simulink model "multi_rotor_sim"  (R2023b)
settings: Solver=ode4  StartTime=0.0  StopTime=inf  FixedStep=ST  RelTol=1e-3
values from neighbouring files (symbols this model uses):
  a0 = 0    [parameters.m]
  ASLOPE = 5.9    [parameters.m]
  Ax = 0.023    [parameters.m]
  Ay = 0.023    [parameters.m]
  Az = 0.106    [parameters.m]
  BLADES = 2    [parameters.m]
  BLCG = 0    [parameters.m]
  BLCP = 0    [parameters.m]
  BLH1 = b*sind(30)    [parameters.m]
  BLH2 = b    (= 0.275)    [parameters.m]
  BLH3 = b*sind(30)    [parameters.m]
  BLH4 = -b*sind(30)    [parameters.m]
  BLH5 = -b    (= -0.275)    [parameters.m]
  BLH6 = -b*sind(30)    [parameters.m]
  chi1 = 1    [parameters.m]
  chi2 = -1    [parameters.m]
  chi3 = 1    [parameters.m]
  chi4 = -1    [parameters.m]
  chi5 = 1    [parameters.m]
  chi6 = -1    [parameters.m]
  CHORD = 17.55e-3    (= 0.01755)    [parameters.m]
  CHORD75 = 21e-3    (= 0.021)    [parameters.m]
  dyn_viscosity = 17.89e-6    (= 1.789e-05)    [parameters.m]
  g0 = 9.80665    [parameters.m]
  href = 0    [parameters.m]
  k_ind = 1.35    [parameters.m]
  k_Omega = 14.92    [parameters.m]
  latref = 44.200626    [parameters.m]
  lonref = 12.063822    [parameters.m]
  m = 2.15    [parameters.m]
  MC_ATT_PITCH = 45*pi/180    (= 0.785398163397)    [parameters.m]
  MC_ATT_ROLL = 45*pi/180    (= 0.785398163397)    [parameters.m]
  MC_PITCH_P = 2    [parameters.m]
  MC_PITCHRATE_D = 0    [parameters.m]
  MC_PITCHRATE_I = 0.05    [parameters.m]
  MC_PITCHRATE_P = 0.09*3    (= 0.27)    [parameters.m]
  MC_RATE_PITCH = 500*pi/180    (= 8.72664625997)    [parameters.m]
  MC_RATE_ROLL = 500*pi/180    (= 8.72664625997)    [parameters.m]
  MC_RATE_YAW = 300*pi/180    (= 5.23598775598)    [parameters.m]
  MC_ROLL_P = 2    [parameters.m]
  MC_ROLLRATE_D = 0    [parameters.m]
  MC_ROLLRATE_I = 0.05    [parameters.m]
  MC_ROLLRATE_P = 0.09*3    (= 0.27)    [parameters.m]
  MC_VEL_FWD = 15    [parameters.m]
  MC_VEL_FWD_OPT = 0.5    [parameters.m]
  MC_VEL_LAT = 15    [parameters.m]
  MC_VEL_LAT_OPT = 0.5    [parameters.m]
  MC_VEL_VERT = 15    [parameters.m]
  MC_YAW_P = 0.55    [parameters.m]
  MC_YAWRATE_D = 0.05    [parameters.m]
  MC_YAWRATE_I = 0.02    [parameters.m]
  MC_YAWRATE_P = 0.15*3    (= 0.45)    [parameters.m]
  MPC_XY_VEL_D_ACC = 0.6    [parameters.m]
  MPC_XY_VEL_I_ACC = 0.8    [parameters.m]
  MPC_XY_VEL_P_ACC = 1.7    [parameters.m]
  MPC_Z_VEL_D_ACC = 0    [parameters.m]
  MPC_Z_VEL_I_ACC = 2    [parameters.m]
  MPC_Z_VEL_P_ACC = 4    [parameters.m]
  n = 0.6359    [parameters.m]
  p00 = 7.145e-2    (= 0.07145)    [parameters.m]
  p01 = 0.4377    [parameters.m]
  p02 = -10.13    [parameters.m]
  p10 = 1.259e-3    (= 0.001259)    [parameters.m]
  p11 = 1.284e-3    (= 0.001284)    [parameters.m]
  p20 = -7.513e-7    (= -7.513e-07)    [parameters.m]
  PWM_hover = (PWM_idle+PWM_max)/2    (= 1550)    [parameters.m]
  PWM_idle = 1100    [parameters.m]
  PWM_max = 2000    [parameters.m]
  ROTOR = 4*0.0254    (= 0.1016)    [parameters.m]
  ST = 0.01    [parameters.m]
  STACG = 0    [parameters.m]
  STACP = 0    [parameters.m]
  STAH1 = -b*cosd(30)    [parameters.m]
  STAH2 = 0    [parameters.m]
  STAH3 = b*cosd(30)    [parameters.m]
  STAH4 = b*cosd(30)    [parameters.m]
  STAH5 = 0    [parameters.m]
  STAH6 = -b*cosd(30)    [parameters.m]
  TERMINAL_SPEED = 0.5    [parameters.m]
  Theta0 = 45*pi/180    (= 0.785398163397)    [parameters.m]
  THETT = -38.0973*pi/180    (= -0.66492332112)    [parameters.m]
  wind_rate = [ 0 0 0 ]'    [parameters.m]
  wind_velocity_e = [ 0 0 0 ]'    [parameters.m]
  WLCG = -0.02    [parameters.m]
  WLCP = -0.08    [parameters.m]
  WLH1 = 32e-3    (= 0.032)    [parameters.m]
  WLH2 = 32e-3    (= 0.032)    [parameters.m]
  WLH3 = 32e-3    (= 0.032)    [parameters.m]
  WLH4 = 32e-3    (= 0.032)    [parameters.m]
  WLH5 = 32e-3    (= 0.032)    [parameters.m]
  WLH6 = 32e-3    (= 0.032)    [parameters.m]
undefined symbols (not defined in the file or in its folder): Earth, WGS84, X, Y, Z
libraries: sm_lib x258, slpidlib x36, nesl_utility x15, sharedtransform x13, aerolibutil x4, aerolibanimutils x3, sharedutil x2, sim3dlib x1, uavsim3dlib x1, shared6dof x1, aerolibtransform2 x1, aerolibatmos2 x1
(part 11 of 11)

== matlab function multi_rotor_sim/MULTIROTOR MODEL/ROTORS FORCE AND MOMENT/ROTOR5/MATLAB Function ==
  data: BLADES input; Mrotor output; ASLOPE input; CHORD input; CHORD75 input; ROTOR input; a0 input; Theta0 input; THETT input; dyn_viscosity input; k_ind input; STACG input; BLCG input; WLCG input; STAH input; BLH input; WLH input; chi input; rho input; TAS input; omega_TAS input; Frotor output; Q output; omega input; Omega input
function [Mrotor,Frotor,Q] = fcn(BLADES,ASLOPE,CHORD,CHORD75,ROTOR,a0,Theta0,THETT,dyn_viscosity,k_ind,STACG,BLCG,WLCG,STAH,BLH,WLH,chi,rho,TAS,omega_TAS,omega,Omega)

%% preliminary calculations
A = pi*ROTOR^2; % area of rotor disc 
sigma = BLADES*CHORD/(pi*ROTOR); % solidity of rotor 
lever_arm_H = [STACG-STAH BLH-BLCG WLCG-WLH]'; % vector from cg to rotor hub
TAS_H = [1 chi 1]'.*(TAS + cross(omega_TAS,lever_arm_H)); % wind speed at rotor
uH = TAS_H(1);
vH = TAS_H(2);
wH = TAS_H(3);
beta_w = atan2(vH,uH); % sideslip angle 
Mu = sqrt(uH^2+vH^2)/(Omega*ROTOR); % advance ratio
p = omega(1); % roll rate
q = omega(2); % pitch rate
pH = chi*p;
qH = q;

%% thrust calculation

lambda = fzero(@(x) x-wH/(Omega*ROTOR)+0.5*((0.5*BLADES*rho*ASLOPE*CHORD*ROTOR*(Omega*ROTOR)^2*(x/2+ ...
         +Theta0*(1/3+Mu^2/2)+THETT*(1/4+Mu^2/4)+Mu/4*(pH/Omega*cos(beta_w)+ ...
         +qH/Omega*sin(beta_w))))/(rho*A*(Omega*ROTOR)^2))/sqrt(Mu^2+x^2), -0.1);
vi = wH-lambda*Omega*ROTOR;
T = (0.5*BLADES*rho*ASLOPE*CHORD*ROTOR*(Omega*ROTOR)^2*(lambda/2+Theta0*(1/3+Mu^2/2)+ ...
    +THETT*(1/4+Mu^2/4)+Mu/4*(pH/Omega*cos(beta_w)+qH/Omega*sin(beta_w))));
CT = T/(rho*A*(Omega*ROTOR)^2);
V75 = sqrt(vi^2+(0.75*(Omega*ROTOR))^2);
Re = rho*CHORD75*V75/dyn_viscosity;
delta = 0.1166*Re^(-0.2)+0.3/ASLOPE^2*(6*CT/sigma/(1+3/2*Mu^2))^2;

%% forces and moments in the hub-wind frame

H_w = BLADES/2*rho*ASLOPE*CHORD*ROTOR*(Omega*ROTOR)^2*(delta*Mu/(2*ASLOPE)-1/4*Theta0*(2*lambda*Mu+ ...
      +2/3*(pH/Omega*cos(beta_w)+qH/Omega*sin(beta_w)))-THETT/4*(Mu*lambda+1/2*(pH/Omega*cos(beta_w)+ ...
      +qH/Omega*sin(beta_w)))+1/4*(-2*a0/3*(-pH/Omega*sin(beta_w)+qH/Omega*cos(beta_w))+ ...
      -2*lambda*(pH/Omega*cos(beta_w)+qH/Omega*sin(beta_w)))+Mu/4*a0^2);
Y_w = BLADES/2*rho*ASLOPE*CHORD*ROTOR*(Omega*ROTOR)^2*(-1/4*Theta0*(3*a0*Mu+ ...
      -2/3*(-pH/Omega*sin(beta_w)+qH/Omega*cos(beta_w)))-THETT/4*(2*a0*Mu+ ...
      -1/2*(-pH/Omega*sin(beta_w)+qH/Omega*cos(beta_w)))-1/4*(2*a0/3*(pH/Omega*cos(beta_w)+ ...
      +qH/Omega*sin(beta_w))-2*lambda*(-pH/Omega*sin(beta_w)+qH/Omega*cos(beta_w)))-Mu/4*6*a0*lambda);
L_w = 0;
M_w = 0;
Q = k_ind*BLADES/2*rho*ASLOPE*CHORD*ROTOR^2*(Omega*ROTOR)^2*(delta/k_ind/(4*ASLOPE)*(1+Mu^2)-Theta0*(lambda/3+ ...
    +Mu/6*(pH/Omega*cos(beta_w)+qH/Omega*sin(beta_w)))-THETT*lambda/4-1/2*lambda^2+ ...
    +Mu/3*a0*(-pH/Omega*sin(beta_w)+qH/Omega*cos(beta_w))-1/8*(-pH/Omega*sin(beta_w)+ ...
    +qH/Omega*cos(beta_w))^2-1/8*(pH/Omega*cos(beta_w)+qH/Omega*sin(beta_w))^2);


%% back rotation from hub_wind frame to hub-frame

H_H = H_w*cos(beta_w)+Y_w*sin(beta_w);
Y_H = -H_w*sin(beta_w)+Y_w*cos(beta_w);
L_H = L_w*cos(beta_w)-M_w*sin(beta_w);
M_H = L_w*sin(beta_w)+M_w*cos(beta_w);

%% back rotation from hub-frame to body-frame

X = -H_H;
Y = chi*Y_H;
Z = -T;
Frotor = [X Y Z]';
Mrotor = [chi*L_H M_H chi*Q]'+cross(lever_arm_H,Frotor);

== matlab function multi_rotor_sim/MULTIROTOR MODEL/ROTORS FORCE AND MOMENT/ROTOR6/ELECTRICAL EFFICIENCY MODEL ==
  data: Q input; Pe output; Omega input; p00 input; p10 input; p01 input; p20 input; p11 input; p02 input
function Pe = fcn(Q,Omega,p00,p10,p01,p20,p11,p02)
eta_e = p00 + p10*Omega + p01*Q + p20*Omega^2 + p02*Q^2 + p11*Omega*Q;
Psh = Omega*Q;
Pe = Psh/eta_e;

== matlab function multi_rotor_sim/MULTIROTOR MODEL/ROTORS FORCE AND MOMENT/ROTOR6/MATLAB Function ==
  data: BLADES input; Mrotor output; ASLOPE input; CHORD input; CHORD75 input; ROTOR input; a0 input; Theta0 input; THETT input; dyn_viscosity input; k_ind input; STACG input; BLCG input; WLCG input; STAH input; BLH input; WLH input; chi input; rho input; TAS input; omega_TAS input; Frotor output; Q output; omega input; Omega input
function [Mrotor,Frotor,Q] = fcn(BLADES,ASLOPE,CHORD,CHORD75,ROTOR,a0,Theta0,THETT,dyn_viscosity,k_ind,STACG,BLCG,WLCG,STAH,BLH,WLH,chi,rho,TAS,omega_TAS,omega,Omega)

%% preliminary calculations
A = pi*ROTOR^2; % area of rotor disc 
sigma = BLADES*CHORD/(pi*ROTOR); % solidity of rotor 
lever_arm_H = [STACG-STAH BLH-BLCG WLCG-WLH]'; % vector from cg to rotor hub
TAS_H = [1 chi 1]'.*(TAS + cross(omega_TAS,lever_arm_H)); % wind speed at rotor
uH = TAS_H(1);
vH = TAS_H(2);
wH = TAS_H(3);
beta_w = atan2(vH,uH); % sideslip angle 
Mu = sqrt(uH^2+vH^2)/(Omega*ROTOR); % advance ratio
p = omega(1); % roll rate
q = omega(2); % pitch rate
pH = chi*p;
qH = q;

%% thrust calculation

lambda = fzero(@(x) x-wH/(Omega*ROTOR)+0.5*((0.5*BLADES*rho*ASLOPE*CHORD*ROTOR*(Omega*ROTOR)^2*(x/2+ ...
         +Theta0*(1/3+Mu^2/2)+THETT*(1/4+Mu^2/4)+Mu/4*(pH/Omega*cos(beta_w)+ ...
         +qH/Omega*sin(beta_w))))/(rho*A*(Omega*ROTOR)^2))/sqrt(Mu^2+x^2), -0.1);
vi = wH-lambda*Omega*ROTOR;
T = (0.5*BLADES*rho*ASLOPE*CHORD*ROTOR*(Omega*ROTOR)^2*(lambda/2+Theta0*(1/3+Mu^2/2)+ ...
    +THETT*(1/4+Mu^2/4)+Mu/4*(pH/Omega*cos(beta_w)+qH/Omega*sin(beta_w))));
CT = T/(rho*A*(Omega*ROTOR)^2);
V75 = sqrt(vi^2+(0.75*(Omega*ROTOR))^2);
Re = rho*CHORD75*V75/dyn_viscosity;
delta = 0.1166*Re^(-0.2)+0.3/ASLOPE^2*(6*CT/sigma/(1+3/2*Mu^2))^2;

%% forces and moments in the hub-wind frame

H_w = BLADES/2*rho*ASLOPE*CHORD*ROTOR*(Omega*ROTOR)^2*(delta*Mu/(2*ASLOPE)-1/4*Theta0*(2*lambda*Mu+ ...
      +2/3*(pH/Omega*cos(beta_w)+qH/Omega*sin(beta_w)))-THETT/4*(Mu*lambda+1/2*(pH/Omega*cos(beta_w)+ ...
      +qH/Omega*sin(beta_w)))+1/4*(-2*a0/3*(-pH/Omega*sin(beta_w)+qH/Omega*cos(beta_w))+ ...
      -2*lambda*(pH/Omega*cos(beta_w)+qH/Omega*sin(beta_w)))+Mu/4*a0^2);
Y_w = BLADES/2*rho*ASLOPE*CHORD*ROTOR*(Omega*ROTOR)^2*(-1/4*Theta0*(3*a0*Mu+ ...
      -2/3*(-pH/Omega*sin(beta_w)+qH/Omega*cos(beta_w)))-THETT/4*(2*a0*Mu+ ...
      -1/2*(-pH/Omega*sin(beta_w)+qH/Omega*cos(beta_w)))-1/4*(2*a0/3*(pH/Omega*cos(beta_w)+ ...
      +qH/Omega*sin(beta_w))-2*lambda*(-pH/Omega*sin(beta_w)+qH/Omega*cos(beta_w)))-Mu/4*6*a0*lambda);
L_w = 0;
M_w = 0;
Q = k_ind*BLADES/2*rho*ASLOPE*CHORD*ROTOR^2*(Omega*ROTOR)^2*(delta/k_ind/(4*ASLOPE)*(1+Mu^2)-Theta0*(lambda/3+ ...
    +Mu/6*(pH/Omega*cos(beta_w)+qH/Omega*sin(beta_w)))-THETT*lambda/4-1/2*lambda^2+ ...
    +Mu/3*a0*(-pH/Omega*sin(beta_w)+qH/Omega*cos(beta_w))-1/8*(-pH/Omega*sin(beta_w)+ ...
    +qH/Omega*cos(beta_w))^2-1/8*(pH/Omega*cos(beta_w)+qH/Omega*sin(beta_w))^2);


%% back rotation from hub_wind frame to hub-frame

H_H = H_w*cos(beta_w)+Y_w*sin(beta_w);
Y_H = -H_w*sin(beta_w)+Y_w*cos(beta_w);
L_H = L_w*cos(beta_w)-M_w*sin(beta_w);
M_H = L_w*sin(beta_w)+M_w*cos(beta_w);

%% back rotation from hub-frame to body-frame

X = -H_H;
Y = chi*Y_H;
Z = -T;
Frotor = [X Y Z]';
Mrotor = [chi*L_H M_H chi*Q]'+cross(lever_arm_H,Frotor);

== matlab function multi_rotor_sim/MULTIROTOR MODEL/ESC+motor/DJI OPTO 3OA + DJI 2212 ==
  data: k_Omega input; Omega_array output; n input; PWM_idle input; PWM_array input
function Omega_array = fcn(k_Omega,n,PWM_idle,PWM_array)
% from tests on DJI OPTO 3OA + DJI 2212, with propeller 8x4.5[in] 
delta = PWM_array-PWM_idle;
Omega_array = k_Omega*delta.^n;

== matlab function multi_rotor_sim/PX4 CONTROL SYSTEM MOD/ACCELERATION AND YAW TO ATTITUDE/MATLAB Function ==
  data: Asp input; theta_sp output; g0 input; psi input; phi_sp output
function [theta_sp,phi_sp] = fcn(Asp,g0,psi)
% step 1: normalization
I_e_cmd_z = (Asp-[0 0 g0]')/(norm(Asp-[0 0 g0]'));
% step 2: first rotation around local z
K_e_cmd_z = [cos(psi) sin(psi) 0; -sin(psi) cos(psi) 0; 0       0       1]*I_e_cmd_z;
% step 3: extraction of remaining two angles 
theta_sp = atan(K_e_cmd_z(1)/K_e_cmd_z(3));
phi_sp = atan(-1/cos(theta_sp)*(K_e_cmd_z(2)*K_e_cmd_z(3))/(K_e_cmd_z(1)^2+K_e_cmd_z(3)^2));

== matlab function multi_rotor_sim/PX4 CONTROL SYSTEM MOD/ATTITUDE CONTROLLER/MATLAB Function ==
  data: qe input; omegasp output; MC_ROLL_P input; MC_PITCH_P input; MC_YAW_P input; yaw_rate_sp input
function omegasp = fcn(qe,MC_ROLL_P,MC_PITCH_P,MC_YAW_P,yaw_rate_sp)
qe0 = qe(1);
qe1 = qe(2);
qe2 = qe(3);
qe3 = qe(4);
if qe0>=0
    s = 1;
else
    s = -1;
end

omegasp = 2*s*[ qe1*MC_ROLL_P, qe2*MC_PITCH_P, qe3*MC_YAW_P ]'+ yaw_rate_sp;

== matlab function multi_rotor_sim/PX4 CONTROL SYSTEM MOD/ATTITUDE MAPPING FROM GCS INPUT/MATLAB Function1 ==
  data: pilot input; eulersp_pilot output; MC_ATT_ROLL input; MC_ATT_PITCH input; MC_RATE_YAW input; psi input; yaw_rate_sp output
function [eulersp_pilot,yaw_rate_sp]  = fcn(pilot,MC_ATT_ROLL,MC_ATT_PITCH,MC_RATE_YAW,psi)

eulersp_pilot = [pilot(2)*MC_ATT_ROLL pilot(3)*MC_ATT_PITCH psi]';
yaw_rate_sp = [ 0 0 MC_RATE_YAW*pilot(4)]';

== matlab function multi_rotor_sim/MULTIROTOR MODEL/ROTORS FORCE AND MOMENT/ROTOR1/ELECTRICAL EFFICIENCY MODEL ==
  data: Q input; Pe output; Omega input; p00 input; p10 input; p01 input; p20 input; p11 input; p02 input
function Pe = fcn(Q,Omega,p00,p10,p01,p20,p11,p02)
eta_e = p00 + p10*Omega + p01*Q + p20*Omega^2 + p02*Q^2 + p11*Omega*Q;
Psh = Omega*Q;
Pe = Psh/eta_e;

== matlab function multi_rotor_sim/PX4 CONTROL SYSTEM MOD/MATLAB Function ==
  data: PWM_vert input; PWM_roll input; PWM_array output; PWM_pitch input; PWM_yaw input
function PWM_array = fcn(PWM_vert,PWM_roll,PWM_pitch,PWM_yaw)

PWM_channels = [PWM_vert,PWM_roll,PWM_pitch,PWM_yaw]';
% MM_matrix = [ 1 -1  1  1 ;
%               1 -1  0 -1 ;
%               1 -1 -1  1 ;
%               1  1 -1 -1 ;
%               1  1  0  1 ;
%               1  1  1 -1 ];
% MM_matrix = [ 1 -1  1  1 ;
%               1 -2  0 -1 ;
%               1 -1 -1  1 ;
%               1  1 -1 -1 ;
%               1  2  0  1 ;
%               1  1  1 -1 ];
MM_matrix = [ 1 -1  sqrt(3)  1 ;
              1 -2    0     -1 ;
              1 -1 -sqrt(3)  1 ;
              1  1 -sqrt(3) -1 ;
              1  2    0      1 ;
              1  1  sqrt(3) -1 ];
PWM_array = MM_matrix*PWM_channels;

== matlab function multi_rotor_sim/PX4 CONTROL SYSTEM MOD/SPEED MAPPING FROM GCS INPUT/MATLAB Function1 ==
  data: pilot input; psi input; Vsp_pilot_inertial output; MC_VEL_FWD input; MC_VEL_LAT input; MC_VEL_VERT input
function Vsp_pilot_inertial = fcn(pilot,psi,MC_VEL_FWD,MC_VEL_LAT,MC_VEL_VERT)

TLE = [cos(psi) sin(psi) 0; -sin(psi) cos(psi) 0; 0       0       1];
Vsp_pilot_local = [-pilot(3)*MC_VEL_FWD pilot(2)*MC_VEL_LAT -pilot(1)*MC_VEL_VERT]';
Vsp_pilot_inertial = TLE'*Vsp_pilot_local;

== matlab function multi_rotor_sim/PX4 CONTROL SYSTEM MOD/VERTICAL CHANNELL CONTROLLER/MATLAB Function ==
  data: Asp input; delta_vert output; g0 input
function delta_vert = fcn(Asp,g0)

delta_vert = -Asp(3)/g0; % basically the load factor

== matlab function multi_rotor_sim/PX4 CONTROL SYSTEM MOD BIS/ACCELERATION AND YAW TO ATTITUDE/MATLAB Function ==
  data: Asp input; theta_sp output; g0 input; psi input; phi_sp output
function [theta_sp,phi_sp] = fcn(Asp,g0,psi)
% step 1: normalization
I_e_cmd_z = (Asp-[0 0 g0]')/(norm(Asp-[0 0 g0]'));
% step 2: first rotation around local z
K_e_cmd_z = [cos(psi) sin(psi) 0; -sin(psi) cos(psi) 0; 0       0       1]*I_e_cmd_z;
% step 3: extraction of remaining two angles 
theta_sp = atan(K_e_cmd_z(1)/K_e_cmd_z(3));
phi_sp = atan(-1/cos(theta_sp)*(K_e_cmd_z(2)*K_e_cmd_z(3))/(K_e_cmd_z(1)^2+K_e_cmd_z(3)^2));

== matlab function multi_rotor_sim/PX4 CONTROL SYSTEM MOD BIS/ANGULAR RATE MAPPING FROM GCS INPUT/MATLAB Function1 ==
  data: pilot input; omegasp_pilot output; MC_RATE_ROLL input; MC_RATE_PITCH input; MC_RATE_YAW input; delta_throttle output
function [omegasp_pilot,delta_throttle]   = fcn(pilot,MC_RATE_ROLL,MC_RATE_PITCH,MC_RATE_YAW)

omegasp_pilot = [pilot(2)*MC_RATE_ROLL pilot(3)*MC_RATE_PITCH MC_RATE_YAW*pilot(4)]';
delta_throttle = pilot(1);

== matlab function multi_rotor_sim/PX4 CONTROL SYSTEM MOD BIS/ATTITUDE CONTROLLER/MATLAB Function ==
  data: qe input; omegasp output; MC_ROLL_P input; MC_PITCH_P input; MC_YAW_P input
function omegasp = fcn(qe,MC_ROLL_P,MC_PITCH_P,MC_YAW_P)
qe0 = qe(1);
qe1 = qe(2);
qe2 = qe(3);
qe3 = qe(4);
if qe0>=0
    s = 1;
else
    s = -1;
end

omegasp = 2*s*[ qe1*MC_ROLL_P, qe2*MC_PITCH_P, qe3*MC_YAW_P ]';

== matlab function multi_rotor_sim/PX4 CONTROL SYSTEM MOD BIS/ATTITUDE MAPPING FROM GCS INPUT/MATLAB Function1 ==
  data: pilot input; eulersp_pilot output; MC_ATT_ROLL input; MC_ATT_PITCH input; psi input
function eulersp_pilot   = fcn(pilot,MC_ATT_ROLL,MC_ATT_PITCH,psi)

eulersp_pilot = [pilot(2)*MC_ATT_ROLL pilot(3)*MC_ATT_PITCH psi]';

== matlab function multi_rotor_sim/PX4 CONTROL SYSTEM MOD BIS/MATLAB Function ==
  data: PWM_vert input; PWM_roll input; PWM_array output; PWM_pitch input; PWM_yaw input
function PWM_array = fcn(PWM_vert,PWM_roll,PWM_pitch,PWM_yaw)

PWM_channels = [PWM_vert,PWM_roll,PWM_pitch,PWM_yaw]';
% MM_matrix = [ 1 -1  1  1 ;
%               1 -1  0 -1 ;
%               1 -1 -1  1 ;
%               1  1 -1 -1 ;
%               1  1  0  1 ;
%               1  1  1 -1 ];
% MM_matrix = [ 1 -1  1  1 ;
%               1 -2  0 -1 ;
%               1 -1 -1  1 ;
%               1  1 -1 -1 ;
%               1  2  0  1 ;
%               1  1  1 -1 ];
MM_matrix = [ 1 -1  sqrt(3)  1 ;
              1 -2    0     -1 ;
              1 -1 -sqrt(3)  1 ;
              1  1 -sqrt(3) -1 ;
              1  2    0      1 ;
              1  1  sqrt(3) -1 ];
PWM_array = MM_matrix*PWM_channels;

== matlab function multi_rotor_sim/PX4 CONTROL SYSTEM MOD/ANGULAR RATE MAPPING FROM GCS INPUT/MATLAB Function1 ==
  data: pilot input; omegasp_pilot output; MC_RATE_ROLL input; MC_RATE_PITCH input; MC_RATE_YAW input; delta_throttle output
function [omegasp_pilot,delta_throttle]   = fcn(pilot,MC_RATE_ROLL,MC_RATE_PITCH,MC_RATE_YAW)

omegasp_pilot = [pilot(2)*MC_RATE_ROLL pilot(3)*MC_RATE_PITCH MC_RATE_YAW*pilot(4)]';
delta_throttle = pilot(1);

== matlab function multi_rotor_sim/PX4 CONTROL SYSTEM MOD/OPTICAL GUIDANCE SYSTEM (PROPORTIONAL LAW)/MATLAB Function ==
  data: centroid_centered input; Vsp_optical output; MC_VEL_FWD input; MC_VEL_LAT input; TERMINAL_SPEED input; psi input
function Vsp_optical= fcn(centroid_centered,MC_VEL_FWD,MC_VEL_LAT,TERMINAL_SPEED,psi)

delta_roll=centroid_centered(1)/320;
delta_pitch=centroid_centered(2)/320;

TLE=[cos(psi) sin(psi) 0;
    -sin(psi) cos(psi) 0;
    0 0 1];

Vsp_optical_local=[MC_VEL_FWD*delta_pitch, MC_VEL_LAT*delta_roll, -TERMINAL_SPEED]';

Vsp_optical=TLE'*Vsp_optical_local;

== matlab function multi_rotor_sim/PX4 CONTROL SYSTEM MOD BIS/SPEED MAPPING FROM GCS INPUT/MATLAB Function1 ==
  data: pilot input; psi input; Vsp_pilot_inertial output; MC_VEL_FWD input; MC_VEL_LAT input; MC_VEL_VERT input
function Vsp_pilot_inertial = fcn(pilot,psi,MC_VEL_FWD,MC_VEL_LAT,MC_VEL_VERT)

TLE = [cos(psi) sin(psi) 0; -sin(psi) cos(psi) 0; 0       0       1];
Vsp_pilot_local = [-pilot(3)*MC_VEL_FWD pilot(2)*MC_VEL_LAT -pilot(1)*MC_VEL_VERT]';
Vsp_pilot_inertial = TLE'*Vsp_pilot_local;

== matlab function multi_rotor_sim/PX4 CONTROL SYSTEM MOD BIS/VERTICAL CHANNELL CONTROLLER/MATLAB Function ==
  data: Asp input; delta_vert output; g0 input
function delta_vert = fcn(Asp,g0)

delta_vert = -Asp(3)/g0; % basically the load factor

== matlab function multi_rotor_sim/MULTIROTOR MODEL/FRAME DRAG FORCE AND MOMENT/FRAME DRAG ==
  data: Ax input; F_frame output; Ay input; Az input; STACP input; BLCP input; WLCP input; STACG input; BLCG input; WLCG input; rho input; TAS input; M_frame output
function [F_frame, M_frame] = fcn(Ax,Ay,Az,STACP,BLCP,WLCP,STACG,BLCG,WLCG,rho,TAS)
lever_arm_cp = [STACG-STACP BLCP-BLCG WLCG-WLCP]';
F_frame = -0.5*rho*[TAS(1)*Ax TAS(2)*Ay TAS(3)*Az]'*norm(TAS);
M_frame = cross(lever_arm_cp,F_frame);

== matlab function multi_rotor_sim/MULTIROTOR MODEL/ROTORS FORCE AND MOMENT/ROTOR1/MATLAB Function ==
  data: BLADES input; Mrotor output; ASLOPE input; CHORD input; CHORD75 input; ROTOR input; a0 input; Theta0 input; THETT input; dyn_viscosity input; k_ind input; STACG input; BLCG input; WLCG input; STAH input; BLH input; WLH input; chi input; rho input; TAS input; omega_TAS input; Frotor output; Q output; omega input; Omega input; vi output
function [Mrotor,Frotor,Q,vi] = fcn(BLADES,ASLOPE,CHORD,CHORD75,ROTOR,a0,Theta0,THETT,dyn_viscosity,k_ind,STACG,BLCG,WLCG,STAH,BLH,WLH,chi,rho,TAS,omega_TAS,omega,Omega)

%% preliminary calculations
A = pi*ROTOR^2; % area of rotor disc 
sigma = BLADES*CHORD/(pi*ROTOR); % solidity of rotor 
lever_arm_H = [STACG-STAH BLH-BLCG WLCG-WLH]'; % vector from cg to rotor hub
TAS_H = [1 chi 1]'.*(TAS + cross(omega_TAS,lever_arm_H)); % wind speed at rotor
uH = TAS_H(1);
vH = TAS_H(2);
wH = TAS_H(3);
beta_w = atan2(vH,uH); % sideslip angle 
Mu = sqrt(uH^2+vH^2)/(Omega*ROTOR); % advance ratio
p = omega(1); % roll rate
q = omega(2); % pitch rate
pH = chi*p;
qH = q;

%% thrust calculation

lambda = fzero(@(x) x-wH/(Omega*ROTOR)+0.5*((0.5*BLADES*rho*ASLOPE*CHORD*ROTOR*(Omega*ROTOR)^2*(x/2+ ...
         +Theta0*(1/3+Mu^2/2)+THETT*(1/4+Mu^2/4)+Mu/4*(pH/Omega*cos(beta_w)+ ...
         +qH/Omega*sin(beta_w))))/(rho*A*(Omega*ROTOR)^2))/sqrt(Mu^2+x^2), -0.1);
vi = wH-lambda*Omega*ROTOR;
T = (0.5*BLADES*rho*ASLOPE*CHORD*ROTOR*(Omega*ROTOR)^2*(lambda/2+Theta0*(1/3+Mu^2/2)+ ...
    +THETT*(1/4+Mu^2/4)+Mu/4*(pH/Omega*cos(beta_w)+qH/Omega*sin(beta_w))));
CT = T/(rho*A*(Omega*ROTOR)^2);
V75 = sqrt(vi^2+(0.75*(Omega*ROTOR))^2);
Re = rho*CHORD75*V75/dyn_viscosity;
delta = 0.1166*Re^(-0.2)+0.3/ASLOPE^2*(6*CT/sigma/(1+3/2*Mu^2))^2;

%% forces and moments in the hub-wind frame

H_w = BLADES/2*rho*ASLOPE*CHORD*ROTOR*(Omega*ROTOR)^2*(delta*Mu/(2*ASLOPE)-1/4*Theta0*(2*lambda*Mu+ ...
      +2/3*(pH/Omega*cos(beta_w)+qH/Omega*sin(beta_w)))-THETT/4*(Mu*lambda+1/2*(pH/Omega*cos(beta_w)+ ...
      +qH/Omega*sin(beta_w)))+1/4*(-2*a0/3*(-pH/Omega*sin(beta_w)+qH/Omega*cos(beta_w))+ ...
      -2*lambda*(pH/Omega*cos(beta_w)+qH/Omega*sin(beta_w)))+Mu/4*a0^2);
Y_w = BLADES/2*rho*ASLOPE*CHORD*ROTOR*(Omega*ROTOR)^2*(-1/4*Theta0*(3*a0*Mu+ ...
      -2/3*(-pH/Omega*sin(beta_w)+qH/Omega*cos(beta_w)))-THETT/4*(2*a0*Mu+ ...
      -1/2*(-pH/Omega*sin(beta_w)+qH/Omega*cos(beta_w)))-1/4*(2*a0/3*(pH/Omega*cos(beta_w)+ ...
      +qH/Omega*sin(beta_w))-2*lambda*(-pH/Omega*sin(beta_w)+qH/Omega*cos(beta_w)))-Mu/4*6*a0*lambda);
L_w = 0;
M_w = 0;
Q = k_ind*BLADES/2*rho*ASLOPE*CHORD*ROTOR^2*(Omega*ROTOR)^2*(delta/k_ind/(4*ASLOPE)*(1+Mu^2)-Theta0*(lambda/3+ ...
    +Mu/6*(pH/Omega*cos(beta_w)+qH/Omega*sin(beta_w)))-THETT*lambda/4-1/2*lambda^2+ ...
    +Mu/3*a0*(-pH/Omega*sin(beta_w)+qH/Omega*cos(beta_w))-1/8*(-pH/Omega*sin(beta_w)+ ...
    +qH/Omega*cos(beta_w))^2-1/8*(pH/Omega*cos(beta_w)+qH/Omega*sin(beta_w))^2);


%% back rotation from hub_wind frame to hub-frame

H_H = H_w*cos(beta_w)+Y_w*sin(beta_w);
Y_H = -H_w*sin(beta_w)+Y_w*cos(beta_w);
L_H = L_w*cos(beta_w)-M_w*sin(beta_w);
M_H = L_w*sin(beta_w)+M_w*cos(beta_w);

%% back rotation from hub-frame to body-frame

X = -H_H;
Y = chi*Y_H;
Z = -T;
Frotor = [X Y Z]';
Mrotor = [chi*L_H M_H chi*Q]'+cross(lever_arm_H,Frotor);

== matlab function multi_rotor_sim/MULTIROTOR MODEL/ROTORS FORCE AND MOMENT/ROTOR2/ELECTRICAL EFFICIENCY MODEL ==
  data: Q input; Pe output; Omega input; p00 input; p10 input; p01 input; p20 input; p11 input; p02 input
function Pe = fcn(Q,Omega,p00,p10,p01,p20,p11,p02)
eta_e = p00 + p10*Omega + p01*Q + p20*Omega^2 + p02*Q^2 + p11*Omega*Q;
Psh = Omega*Q;
Pe = Psh/eta_e;
